simulink model "PID_Drone"  (R2021a)
settings: Solver=VariableStepAuto  StartTime=0.0  StopTime=20  RelTol=1e-3
values from neighbouring files (symbols this model uses):
  armLength = 0.046    [droneParameters.m]
  attitudeInit = [0;0;0]    [droneParameters.m]
  dragConstant = 1.368e-10    [droneParameters.m]
  g = 9.81    [droneParameters.m]
  I = diag([Ix, Iy, Iz])    [droneParameters.m]
  ks = 900.5899    [droneParameters.m]
  m = 0.023    [droneParameters.m]
  MotorSpeedInit = [0;0;0]    [droneParameters.m]
  omegaInit = [0;0;0]    [droneParameters.m]
  pKd = 2 * s * w * Ix    (= 0.000383216)    [droneParameters.m]
  pKp = w^2 * Ix / pKd    (= 6.25)    [droneParameters.m]
  posInit = [0;0;0]    [droneParameters.m]
  sKd = 2 * s * w * Iz    (= 0.000388164)    [droneParameters.m]
  sKp = w^2 * Iz / sKd    (= 8.33333333333)    [droneParameters.m]
  tau = 1/10    (= 0.1)    [droneParameters.m]
  thrustConstant = 2.23e-8    (= 2.23e-08)    [droneParameters.m]
  tKd = 2 * s * w * Iy    (= 0.000287412)    [droneParameters.m]
  tKp = w^2 * Iy / tKd    (= 8.33333333333)    [droneParameters.m]
  velInit = [0;0;0]    [droneParameters.m]
  xKd = 2 * s * w * m    (= 0.0644)    [droneParameters.m]
  xKp = w^2 * m / xKd    (= 1.42857142857)    [droneParameters.m]
  yKd = 2 * s * w * m    (= 0.0644)    [droneParameters.m]
  yKp = w^2 * m / yKd    (= 1.42857142857)    [droneParameters.m]
  zKd = 2 * s * w * m    (= 0.0552)    [droneParameters.m]
  zKp = w^2 * m / zKd    (= 1.66666666667)    [droneParameters.m]
libraries: dspstat3 x3
settings Model: Creator=Viet Do  LastModifiedBy=Viet Do

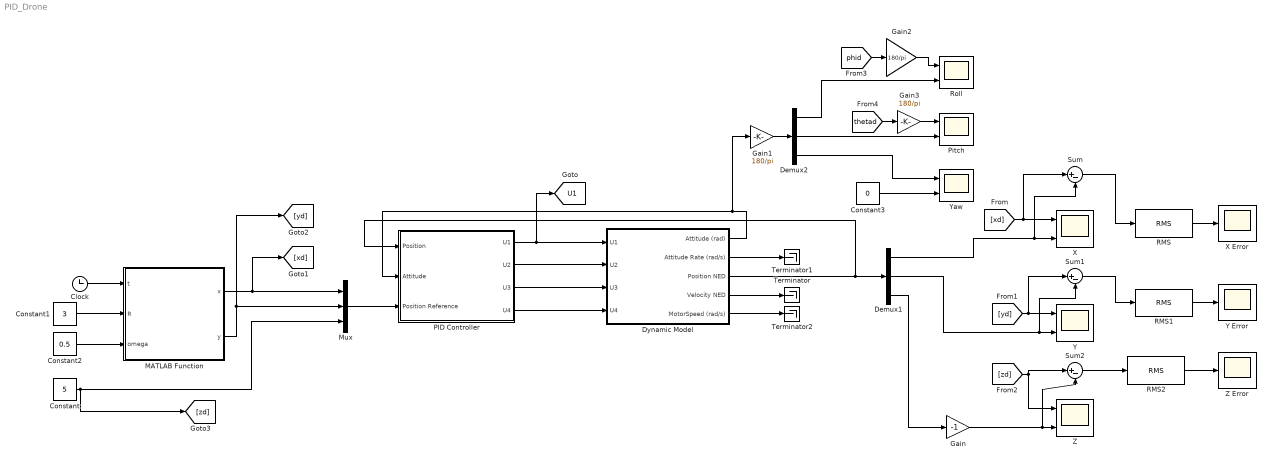
== system PID_Drone ==
  Clock : Clock
  Constant : Constant  Value=5
  Constant1 : Constant  Value=3
  Constant2 : Constant  Value=0.5
  Constant3 : Constant  Value=0
  Demux1 : Demux  Outputs=3
  Demux2 : Demux  Outputs=3
  Dynamic Model : Subsystem
  Gain : Gain  Gain=-1
  Gain1 : Gain  Gain=180/pi
  Gain2 : Gain  Gain=180/pi
  Gain3 : Gain  Gain=180/pi
  MATLAB Function : MATLAB Function  TreatAsAtomicUnit=on
  Mux : Mux  Inputs=3
  PID Controller : Subsystem
  Pitch : Scope  NumInputPorts=2
  RMS : dspstat3/RMS  run=off  directionMode=Each column  dimension=1  InputProcessing=Columns as channels (frame based)  reset_popup=None
  RMS1 : dspstat3/RMS  run=off  directionMode=Each column  dimension=1  InputProcessing=Columns as channels (frame based)  reset_popup=None
  RMS2 : dspstat3/RMS  run=off  directionMode=Each column  dimension=1  InputProcessing=Columns as channels (frame based)  reset_popup=None
  Roll : Scope  NumInputPorts=2
  Sum : Sum  Inputs=|+-
  Sum1 : Sum  Inputs=|+-
  Sum2 : Sum  Inputs=|+-
  Terminator : Terminator
  Terminator1 : Terminator
  Terminator2 : Terminator
  X : Scope  NumInputPorts=2
  X Error : Scope
  Y : Scope  NumInputPorts=2
  Y Error : Scope
  Yaw : Scope  NumInputPorts=2
  Z : Scope  NumInputPorts=2
  Z Error : Scope
  tag scope: U1=global
  wires:
  Clock/1 -> MATLAB Function/1(t)
  Constant2/1 -> MATLAB Function/3(omega)
  Constant1/1 -> MATLAB Function/2(R)
  Mux/1 -> PID Controller/3(Position Reference)
  MATLAB Function/1(x) -> [xd], Mux/1
  PID Controller/1(U1) -> [U1], Dynamic Model/1(U1)
  PID Controller/2(U2) -> Dynamic Model/2(U2)
  PID Controller/3(U3) -> Dynamic Model/3(U3)
  PID Controller/4(U4) -> Dynamic Model/4(U4)
  MATLAB Function/2(y) -> [yd], Mux/2
  Dynamic Model/4(Velocity NED) -> Terminator/1
  Dynamic Model/2(Attitude Rate (rad/s)) -> Terminator1/1
  Dynamic Model/5(MotorSpeed (rad/s)) -> Terminator2/1
  Constant/1 -> [zd], Mux/3
  Gain/1 -> Sum2/2, Z/2
  [xd] -> Sum/1, X/1
  Demux1/1 -> Sum/2, X/2
  [yd] -> Sum1/1, Y/1
  Dynamic Model/3(Position NED) -> Demux1/1, PID Controller/1(Position)
  [zd] -> Z/1, Sum2/1
  Demux1/2 -> Sum1/2, Y/2
  Demux1/3 -> Gain/1
  RMS/1 -> X Error/1
  Sum/1 -> RMS/1
  RMS2/1 -> Z Error/1
  RMS1/1 -> Y Error/1
  Sum1/1 -> RMS1/1
  Sum2/1 -> RMS2/1
  Gain1/1 -> Demux2/1
  Dynamic Model/1(Attitude (rad)) -> Gain1/1, PID Controller/2(Attitude)
  Demux2/1 -> Roll/2
  Gain3/1 -> Pitch/1
  Demux2/2 -> Pitch/2
  Demux2/3 -> Yaw/1
  [thetad] -> Gain3/1
  Gain2/1 -> Roll/1
  [phid] -> Gain2/1
  Constant3/1 -> Yaw/2

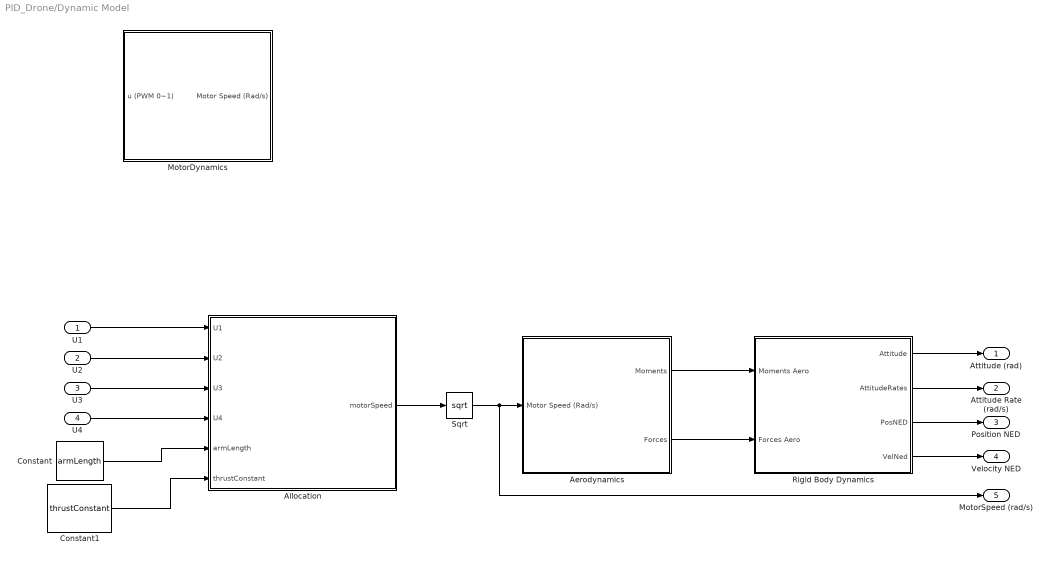
== system PID_Drone/Dynamic Model ==
  U1 : Inport
  U2 : Inport  Port=2
  U3 : Inport  Port=3
  U4 : Inport  Port=4
  Aerodynamics : Subsystem
  Allocation : MATLAB Function  TreatAsAtomicUnit=on
  Constant : Constant  Value=armLength
  Constant1 : Constant  Value=thrustConstant
  MotorDynamics : Subsystem
  Rigid Body Dynamics : Subsystem
  Sqrt : Sqrt  SaturateOnIntegerOverflow=on
  Attitude (rad) : Outport
  Attitude Rate (rad/s) : Outport  Port=2
  Position NED : Outport  Port=3
  Velocity NED : Outport  Port=4
  MotorSpeed (rad/s) : Outport  Port=5
  wires:
  Aerodynamics/2(Forces) -> Rigid Body Dynamics/2(Forces Aero)
  Aerodynamics/1(Moments) -> Rigid Body Dynamics/1(Moments Aero)
  U4/1 -> Allocation/4(U4)
  U3/1 -> Allocation/3(U3)
  U2/1 -> Allocation/2(U2)
  U1/1 -> Allocation/1(U1)
  Rigid Body Dynamics/1(Attitude) -> Attitude (rad)/1
  Rigid Body Dynamics/2(AttitudeRates) -> Attitude Rate (rad/s)/1
  Rigid Body Dynamics/3(PosNED) -> Position NED/1
  Rigid Body Dynamics/4(VelNed) -> Velocity NED/1
  Allocation/1(motorSpeed) -> Sqrt/1
  Sqrt/1 -> MotorSpeed (rad/s)/1, Aerodynamics/1(Motor Speed (Rad/s))
  Constant/1 -> Allocation/5(armLength)
  Constant1/1 -> Allocation/6(thrustConstant)

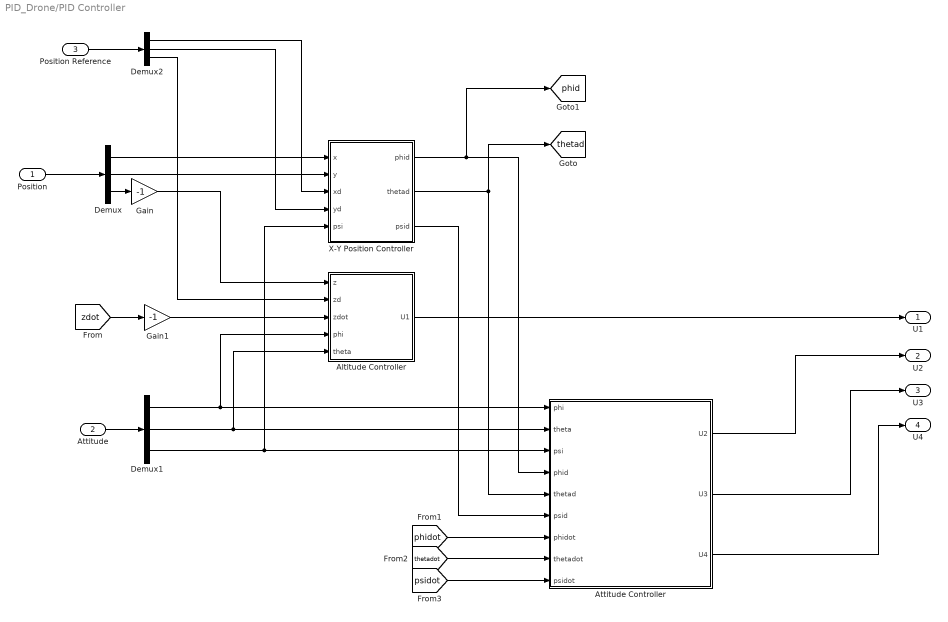
== system PID_Drone/PID Controller ==
  Position : Inport
  Attitude : Inport  Port=2
  Position Reference : Inport  Port=3
  Altitude Controller : Subsystem
  Attitude Controller : Subsystem
  Demux : Demux  Outputs=3
  Demux1 : Demux  Outputs=3
  Demux2 : Demux  Outputs=3
  Gain : Gain  Gain=-1
  Gain1 : Gain  Gain=-1
  X-Y Position Controller : Subsystem
  U1 : Outport
  U2 : Outport  Port=2
  U3 : Outport  Port=3
  U4 : Outport  Port=4
  tag scope: phid=global, thetad=global
  wires:
  Position/1 -> Demux/1
  Attitude/1 -> Demux1/1
  Demux/1 -> X-Y Position Controller/1(x)
  Demux/2 -> X-Y Position Controller/2(y)
  Position Reference/1 -> Demux2/1
  Demux2/1 -> X-Y Position Controller/3(xd)
  Demux2/2 -> X-Y Position Controller/4(yd)
  X-Y Position Controller/3(psid) -> Attitude Controller/6(psid)
  Demux1/1 -> Altitude Controller/4(phi), Attitude Controller/1("phi ")
  Demux1/2 -> Altitude Controller/5(theta), Attitude Controller/2(theta)
  Demux1/3 -> X-Y Position Controller/5(psi), Attitude Controller/3(psi)
  Attitude Controller/1(U2) -> U2/1
  Attitude Controller/2(U3) -> U3/1
  Attitude Controller/3(U4) -> U4/1
  Altitude Controller/1(U1) -> U1/1
  Demux2/3 -> Altitude Controller/2(zd)
  [zdot] -> Gain1/1
  [phidot] -> Attitude Controller/7(phidot)
  [thetadot] -> Attitude Controller/8(thetadot)
  [psidot] -> Attitude Controller/9(psidot)
  Demux/3 -> Gain/1
  Gain/1 -> Altitude Controller/1(z)
  Gain1/1 -> Altitude Controller/3(zdot)
  X-Y Position Controller/2(thetad) -> [thetad], Attitude Controller/5(thetad)
  X-Y Position Controller/1(phid) -> [phid], Attitude Controller/4(phid)

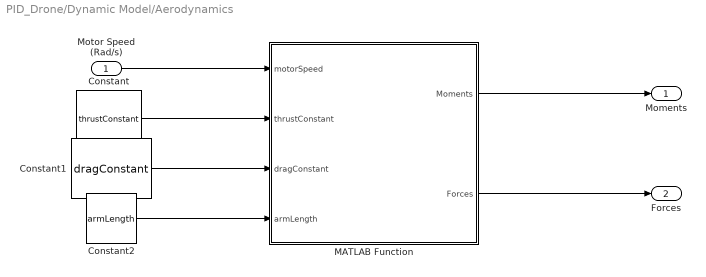
== system PID_Drone/Dynamic Model/Aerodynamics ==
  Motor Speed (Rad/s) : Inport
  Constant : Constant  Value=thrustConstant
  Constant1 : Constant  Value=dragConstant
  Constant2 : Constant  Value=armLength
  MATLAB Function : MATLAB Function  TreatAsAtomicUnit=on
  Moments : Outport
  Forces : Outport  Port=2
  wires:
  MATLAB Function/1(Moments) -> Moments/1
  MATLAB Function/2(Forces) -> Forces/1
  Motor Speed (Rad/s)/1 -> MATLAB Function/1(motorSpeed)
  Constant/1 -> MATLAB Function/2(thrustConstant)
  Constant2/1 -> MATLAB Function/4(armLength)
  Constant1/1 -> MATLAB Function/3(dragConstant)

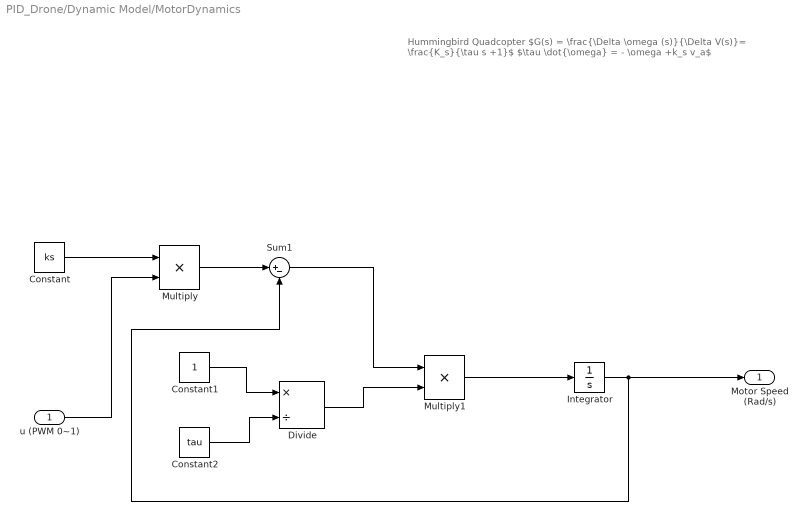
== system PID_Drone/Dynamic Model/MotorDynamics ==
  note: Hummingbird Quadcopter
      | $G(s) = \frac{\Delta \omega (s)}{\Delta V(s)}= \frac{K_s}{\tau s +1}$
      | $\tau \dot{\omega} = - \omega +k_s v_a$
  u (PWM 0~1) : Inport
  Constant : Constant  Value=ks
  Constant1 : Constant
  Constant2 : Constant  Value=tau
  Divide : Product  Inputs=*/
  Integrator : Integrator  InitialCondition=MotorSpeedInit
  Multiply : Product
  Multiply1 : Product
  Sum1 : Sum  Inputs=|+-
  Motor Speed (Rad/s) : Outport
  wires:
  Integrator/1 -> Motor Speed (Rad/s)/1, Sum1/2
  Constant/1 -> Multiply/1
  u (PWM 0~1)/1 -> Multiply/2
  Multiply/1 -> Sum1/1
  Constant1/1 -> Divide/1
  Constant2/1 -> Divide/2
  Sum1/1 -> Multiply1/1
  Multiply1/1 -> Integrator/1
  Divide/1 -> Multiply1/2

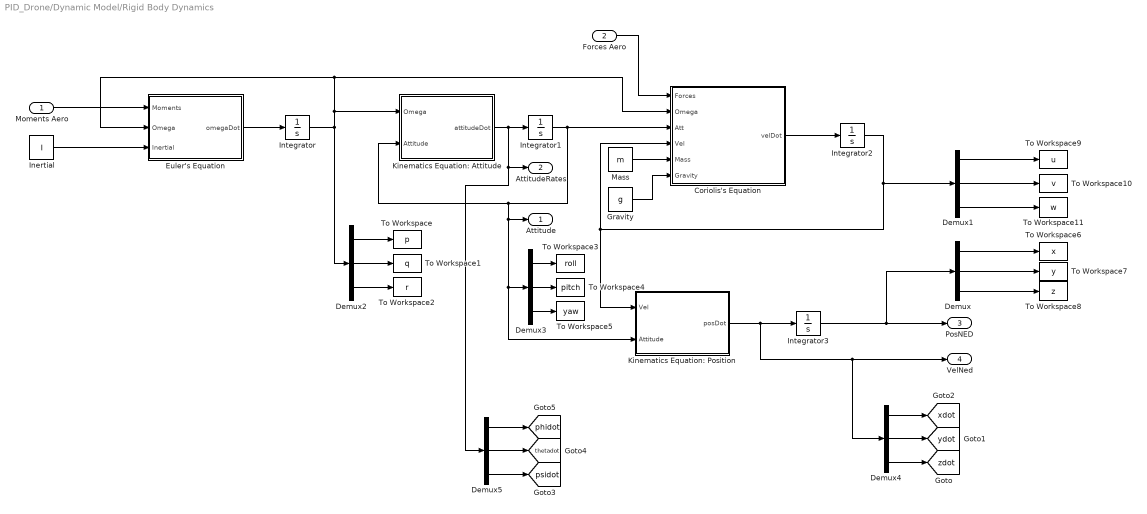
== system PID_Drone/Dynamic Model/Rigid Body Dynamics ==
  Moments Aero : Inport
  Forces Aero : Inport  Port=2
  Coriolis's Equation : MATLAB Function  TreatAsAtomicUnit=on
  Demux{,1..5} (6 alike) : Demux  Outputs=3
  Euler's Equation : MATLAB Function  TreatAsAtomicUnit=on
  Gravity : Constant  Value=g
  Inertial : Constant  Value=I
  Integrator : Integrator  InitialCondition=omegaInit
  Integrator1 : Integrator  InitialCondition=attitudeInit
  Integrator2 : Integrator  InitialCondition=velInit
  Integrator3 : Integrator  InitialCondition=posInit
  Kinematics Equation: Attitude : MATLAB Function  TreatAsAtomicUnit=on
  Kinematics Equation: Position : MATLAB Function  TreatAsAtomicUnit=on
  Mass : Constant  Value=m
  To Workspace : ToWorkspace  VariableName=p  SampleTime=-1
      settings: Save2DSignal=2-D array (concatenate along first dimension)
  To Workspace1 : ToWorkspace  VariableName=q  SampleTime=-1
      settings: Save2DSignal=2-D array (concatenate along first dimension)
  To Workspace10 : ToWorkspace  VariableName=v  SampleTime=-1
      settings: Save2DSignal=2-D array (concatenate along first dimension)
  To Workspace11 : ToWorkspace  VariableName=w  SampleTime=-1
      settings: Save2DSignal=2-D array (concatenate along first dimension)
  To Workspace2 : ToWorkspace  VariableName=r  SampleTime=-1
      settings: Save2DSignal=2-D array (concatenate along first dimension)
  To Workspace3 : ToWorkspace  VariableName=roll  SampleTime=-1
      settings: Save2DSignal=2-D array (concatenate along first dimension)
  To Workspace4 : ToWorkspace  VariableName=pitch  SampleTime=-1
      settings: Save2DSignal=2-D array (concatenate along first dimension)
  To Workspace5 : ToWorkspace  VariableName=yaw  SampleTime=-1
      settings: Save2DSignal=2-D array (concatenate along first dimension)
  To Workspace6 : ToWorkspace  VariableName=x  SampleTime=-1
      settings: Save2DSignal=2-D array (concatenate along first dimension)
  To Workspace7 : ToWorkspace  VariableName=y  SampleTime=-1
      settings: Save2DSignal=2-D array (concatenate along first dimension)
  To Workspace8 : ToWorkspace  VariableName=z  SampleTime=-1
      settings: Save2DSignal=2-D array (concatenate along first dimension)
  To Workspace9 : ToWorkspace  VariableName=u  SampleTime=-1
      settings: Save2DSignal=2-D array (concatenate along first dimension)
  Attitude : Outport
  AttitudeRates : Outport  Port=2
  PosNED : Outport  Port=3
  VelNed : Outport  Port=4
  tag scope: phidot=global, psidot=global, thetadot=global, xdot=global, ydot=global, zdot=global
  wires:
  Moments Aero/1 -> Euler's Equation/1(Moments)
  Inertial/1 -> Euler's Equation/3(Inertial)
  Euler's Equation/1(omegaDot) -> Integrator/1
  Integrator/1 -> Euler's Equation/2(Omega), Coriolis's Equation/2(Omega), Kinematics Equation: Attitude/1(Omega), Demux2/1
  Integrator1/1 -> Coriolis's Equation/3(Att), Kinematics Equation: Attitude/2(Attitude), Demux3/1, Kinematics Equation: Position/2(Attitude), Attitude/1
  Coriolis's Equation/1(velDot) -> Integrator2/1
  Integrator2/1 -> Coriolis's Equation/4(Vel), Kinematics Equation: Position/1(Vel), Demux1/1
  Gravity/1 -> Coriolis's Equation/6(Gravity)
  Mass/1 -> Coriolis's Equation/5(Mass)
  Forces Aero/1 -> Coriolis's Equation/1(Forces)
  Kinematics Equation: Position/1(posDot) -> Demux4/1, VelNed/1, Integrator3/1
  Integrator3/1 -> Demux/1, PosNED/1
  Demux2/1 -> To Workspace/1
  Demux2/2 -> To Workspace1/1
  Demux2/3 -> To Workspace2/1
  Demux3/1 -> To Workspace3/1
  Demux3/2 -> To Workspace4/1
  Demux3/3 -> To Workspace5/1
  Demux/1 -> To Workspace6/1
  Demux/2 -> To Workspace7/1
  Demux/3 -> To Workspace8/1
  Demux1/1 -> To Workspace9/1
  Demux1/2 -> To Workspace10/1
  Demux1/3 -> To Workspace11/1
  Demux4/3 -> [zdot]
  Demux4/2 -> [ydot]
  Demux4/1 -> [xdot]
  Demux5/3 -> [psidot]
  Demux5/1 -> [phidot]
  Demux5/2 -> [thetadot]
  Kinematics Equation: Attitude/1(attitudeDot) -> Demux5/1, AttitudeRates/1, Integrator1/1

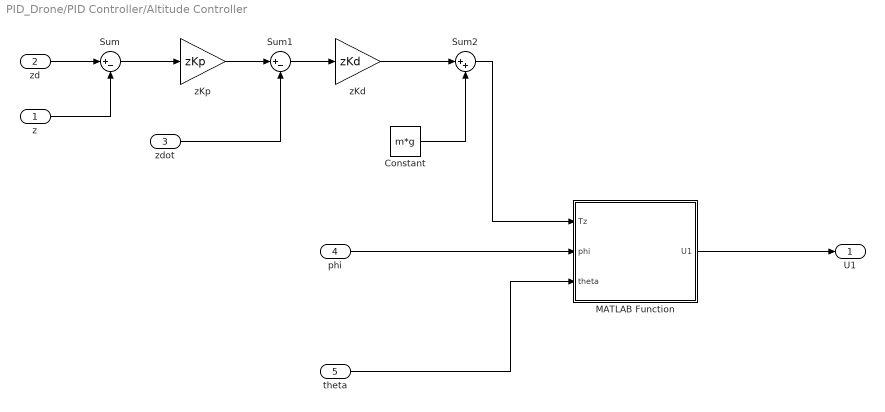
== system PID_Drone/PID Controller/Altitude Controller ==
  z : Inport
  zd : Inport  Port=2
  zdot : Inport  Port=3
  phi : Inport  Port=4
  theta : Inport  Port=5
  Constant : Constant  Value=m*g
  MATLAB Function : MATLAB Function  TreatAsAtomicUnit=on
  Sum : Sum  Inputs=|+-
  Sum1 : Sum  Inputs=|+-
  Sum2 : Sum  Inputs=|++
  zKd : Gain  Gain=zKd
  zKp : Gain  Gain=zKp
  U1 : Outport
  wires:
  MATLAB Function/1(U1) -> U1/1
  phi/1 -> MATLAB Function/2(phi)
  theta/1 -> MATLAB Function/3(theta)
  Sum/1 -> zKp/1
  zdot/1 -> Sum1/2
  Sum2/1 -> MATLAB Function/1(Tz)
  zKp/1 -> Sum1/1
  Sum1/1 -> zKd/1
  zKd/1 -> Sum2/1
  Constant/1 -> Sum2/2
  z/1 -> Sum/2
  zd/1 -> Sum/1

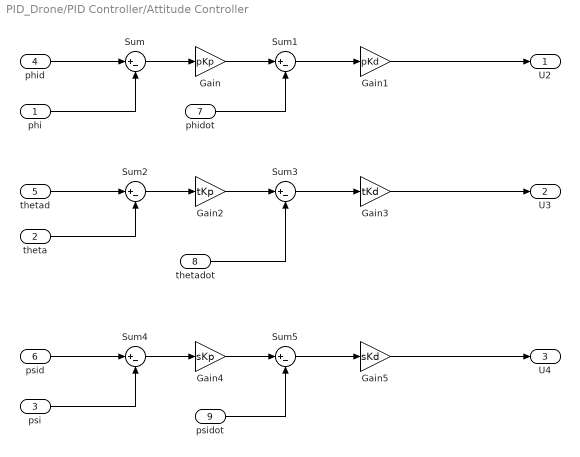
== system PID_Drone/PID Controller/Attitude Controller ==
  "phi " : Inport
  theta : Inport  Port=2
  psi : Inport  Port=3
  phid : Inport  Port=4
  thetad : Inport  Port=5
  psid : Inport  Port=6
  phidot : Inport  Port=7
  thetadot : Inport  Port=8
  psidot : Inport  Port=9
  Gain : Gain  Gain=pKp
  Gain1 : Gain  Gain=pKd
  Gain2 : Gain  Gain=tKp
  Gain3 : Gain  Gain=tKd
  Gain4 : Gain  Gain=sKp
  Gain5 : Gain  Gain=sKd
  Sum{,1..5} (6 alike) : Sum  Inputs=|+-
  U2 : Outport
  U3 : Outport  Port=2
  U4 : Outport  Port=3
  wires:
  Sum/1 -> Gain/1
  Gain/1 -> Sum1/1
  phidot/1 -> Sum1/2
  Sum1/1 -> Gain1/1
  Gain1/1 -> U2/1
  Sum2/1 -> Gain2/1
  Gain2/1 -> Sum3/1
  thetadot/1 -> Sum3/2
  Sum3/1 -> Gain3/1
  Gain3/1 -> U3/1
  Sum4/1 -> Gain4/1
  Gain4/1 -> Sum5/1
  Sum5/1 -> Gain5/1
  Gain5/1 -> U4/1
  psidot/1 -> Sum5/2
  phid/1 -> Sum/1
  "phi "/1 -> Sum/2
  thetad/1 -> Sum2/1
  theta/1 -> Sum2/2
  psid/1 -> Sum4/1
  psi/1 -> Sum4/2

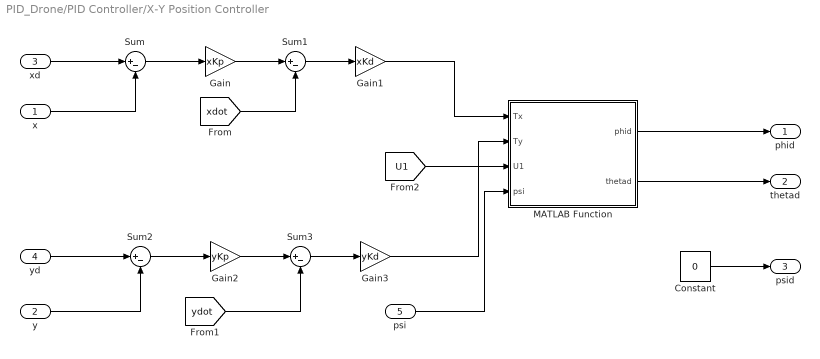
== system PID_Drone/PID Controller/X-Y Position Controller ==
  x : Inport
  y : Inport  Port=2
  xd : Inport  Port=3
  yd : Inport  Port=4
  psi : Inport  Port=5
  Constant : Constant  Value=0
  Gain : Gain  Gain=xKp
  Gain1 : Gain  Gain=xKd
  Gain2 : Gain  Gain=yKp
  Gain3 : Gain  Gain=yKd
  MATLAB Function : MATLAB Function  TreatAsAtomicUnit=on
  Sum{,1..3} (4 alike) : Sum  Inputs=|+-
  phid : Outport
  thetad : Outport  Port=2
  psid : Outport  Port=3
  wires:
  Sum/1 -> Gain/1
  Gain/1 -> Sum1/1
  [xdot] -> Sum1/2
  Sum1/1 -> Gain1/1
  [ydot] -> Sum3/2
  Sum3/1 -> Gain3/1
  Gain2/1 -> Sum3/1
  Sum2/1 -> Gain2/1
  MATLAB Function/1(phid) -> phid/1
  MATLAB Function/2(thetad) -> thetad/1
  Gain1/1 -> MATLAB Function/1(Tx)
  Gain3/1 -> MATLAB Function/2(Ty)
  psi/1 -> MATLAB Function/4(psi)
  [U1] -> MATLAB Function/3(U1)
  Constant/1 -> psid/1
  xd/1 -> Sum/1
  x/1 -> Sum/2
  yd/1 -> Sum2/1
  y/1 -> Sum2/2

== matlab function PID_Drone/Dynamic Model/Rigid Body Dynamics/Kinematics Equation: Attitude ==
  data: Omega input; attitudeDot output; Attitude input
function attitudeDot = fcn(Omega, Attitude)

    p = Attitude(1);
    t = Attitude(2);
    
    Jinv = [1, sin(p) * tan(t), cos(p) * tan(t);...
               0,     cos(p)       ,     -sin(p);...
               0, sin(p)/cos(t) , cos(p)/cos(t)];
    
    attitudeDot = Jinv * Omega;

end

== matlab function PID_Drone/Dynamic Model/Rigid Body Dynamics/Euler's Equation ==
  data: Moments input; omegaDot output; Omega input; Inertial input
function omegaDot = fcn(Moments, Omega, Inertial)

    omegaDot = Inertial^(-1) * (Moments - cross(Omega, Inertial * Omega));

end

== matlab function PID_Drone/Dynamic Model/Rigid Body Dynamics/Coriolis's Equation ==
  data: Forces input; velDot output; Omega input; Att input; Vel input; Mass input; Gravity input
function velDot = fcn(Forces, Omega, Att, Vel, Mass, Gravity)
    
    p = Att(1);
    t = Att(2);
    
    g = [-sin(t);...
            sin(p) * cos(t);...
            cos(p) * cos(t)] * Gravity;
        
    velDot = 1 / Mass * Forces + g - cross(Omega, Vel);

end

== matlab function PID_Drone/Dynamic Model/Rigid Body Dynamics/Kinematics Equation: Position ==
  data: Vel input; posDot output; Attitude input
function posDot = fcn(Vel, Attitude)

    p = Attitude(1);
    t = Attitude(2);
    s = Attitude(3);

    R = [cos(t) * cos(s), sin(p) * sin(t) * cos(s) - cos(p) * sin(s), cos(p) * sin(t) * cos(s) + sin(p) * sin(s); ...
           cos(t) * sin(s), sin(p) * sin(t) * sin(s) + cos(p) * cos(s), cos(p) * sin(t) * sin(s) - sin(p) * cos(s);...
           -sin(t), sin(p) * cos(t), cos(p) * cos(t)];
    
    posDot = R * Vel;
    
end

== matlab function PID_Drone/Dynamic Model/Aerodynamics/MATLAB Function ==
  data: motorSpeed input; Moments output; Forces output; thrustConstant input; dragConstant input; armLength input
function [Moments, Forces] = fcn(motorSpeed, thrustConstant, dragConstant, armLength)
        
        drag = dragConstant * motorSpeed.^2;
        U1 = sum(thrustConstant * motorSpeed.^2);
        
        U2 = sqrt(2) / 2 * armLength * thrustConstant * (motorSpeed(3).^2 + motorSpeed(4).^2 - motorSpeed(1).^2 - motorSpeed(2).^2);
        U3 = sqrt(2) / 2 * armLength * thrustConstant * (motorSpeed(1).^2 + motorSpeed(4).^2 - motorSpeed(2).^2 - motorSpeed(3).^2);
        U4 = drag(1) - drag(2) + drag(3) - drag(4);
        
        Forces = [0; 0; -U1];
        Moments = [U2; U3; U4];
        
end

== matlab function PID_Drone/MATLAB Function ==
  data: x output; t input; y output; R input; omega input
function [x,y] = fcn(t, R, omega)
%     x = R * sin(omega * t);
%     y = R * cos(omega * t);

    if t < 10
        x = 0;
    else
        x = 3;
    end
    y=0;
end

== matlab function PID_Drone/PID Controller/Altitude Controller/MATLAB Function ==
  data: Tz input; U1 output; phi input; theta input
function U1 = fcn(Tz, phi, theta)

    U1 = Tz / (cos(phi) * cos(theta));

end

== matlab function PID_Drone/Dynamic Model/Allocation ==
  data: U1 input; motorSpeed output; U2 input; U3 input; U4 input; armLength input; thrustConstant input
function motorSpeed = fcn(U1, U2, U3, U4, armLength, thrustConstant)

a = 1/(4 * thrustConstant);
b = sqrt(2) / (4 * armLength * thrustConstant);

motorSpeed =  [a, -b, b, a; ...
                         a, -b, -b, -a; ...
                         a, b, -b, a; ...
                         a, b, b, -a] * [U1; U2; U3; U4];

end

== matlab function PID_Drone/PID Controller/X-Y Position Controller/MATLAB Function ==
  data: Tx input; phid output; Ty input; U1 input; psi input; thetad output
function [phid, thetad] = fcn(Tx, Ty, U1, psi)

    if U1 == 0
        phid = 0;
        thetad = 0;
    else
        phid = (-Tx * sin(psi) + Ty * cos(psi)) / U1;
        thetad = -(Tx * cos(psi) + Ty * sin(psi)) / U1;
    end
    
end
